simulink model "Final_proj"  (R2019a)
settings: Solver=VariableStepAuto  StartTime=0.0  StopTime=300  RelTol=1e-3
undefined symbols (not defined in the file): A, b, B, c, F, KI_, KT, KT_
settings Model: Creator=agtaye  LastModifiedBy=agtaye

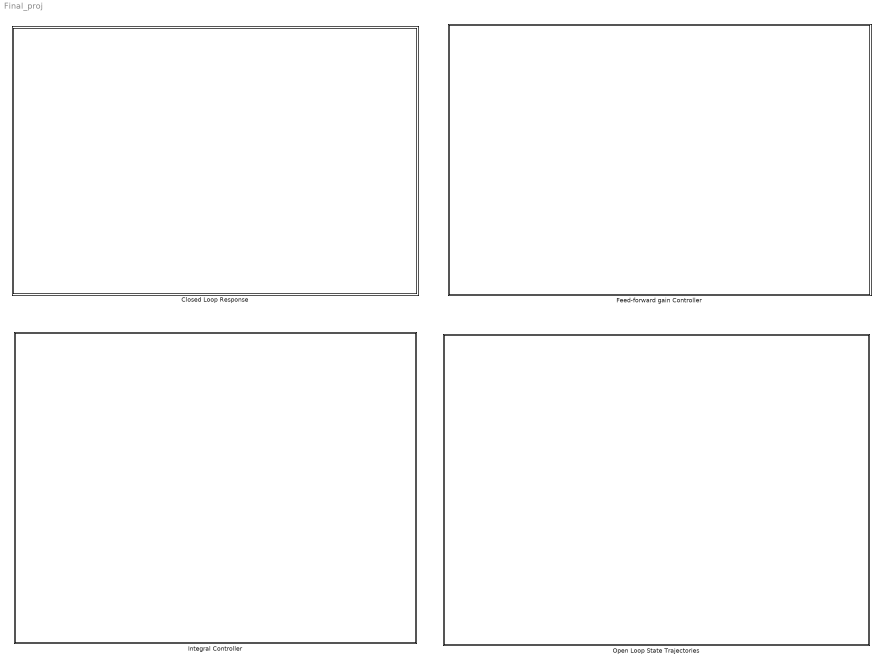
== system Final_proj ==
  Closed Loop Response : Subsystem
  Feed-forward gain Controller : Subsystem
  Integral Controller : Subsystem
  Open Loop State Trajectories : Subsystem

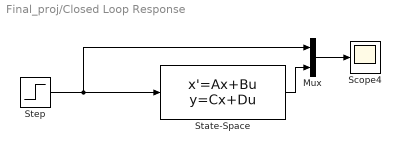
== system Final_proj/Closed Loop Response ==
  Mux : Mux  Inputs=2
  Scope4 : Scope
  State-Space : StateSpace  A="[0\t1\t0\t0; 63.7929491356160\t-5.61041746387390\t-70.7129377085583\t5.60838779731902; 46.9375000000000\t0\t-48.1712500000000\t1; 2182.58450488262\t-49.4418039003888\t-2245.08904324417\t50.6576674638739]"  B=[0;0.0006;0;0.0056]  C=[0 0 1 0]  D=0  InitialCondition=0
  Step : Step  Time=0  After=2  SampleTime=0
  wires:
  Mux/1 -> Scope4/1
  Step/1 -> Mux/1, State-Space/1
  State-Space/1 -> Mux/2

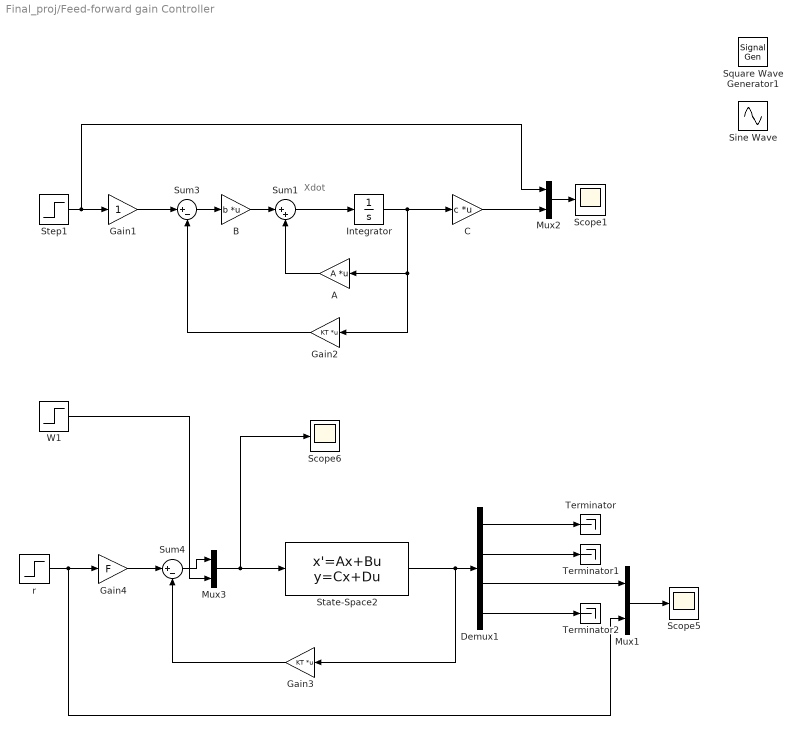
== system Final_proj/Feed-forward gain Controller ==
  note: Xdot
  A : Gain  Gain=A  Multiplication=Matrix(K*u)
  B : Gain  Gain=b  Multiplication=Matrix(K*u)
  "C " : Gain  Gain=c  Multiplication=Matrix(K*u)
  Demux1 : Demux
  Gain1 : Gain
  Gain2 : Gain  Gain=KT  Multiplication=Matrix(K*u)
  Gain3 : Gain  Gain=KT  Multiplication=Matrix(K*u)
  Gain4 : Gain  Gain=F
  Integrator : Integrator
  Mux1 : Mux  Inputs=2
  Mux2 : Mux  Inputs=2
  Mux3 : Mux  Inputs=2
  Scope1 : Scope
  Scope5 : Scope
  Scope6 : Scope
  Sine Wave : Sin  Amplitude=0.00001  Frequency=0.05  SampleTime=0
  Square Wave Generator1 : SignalGenerator  WaveForm=square  Amplitude=0.00001  Frequency=0.05  Units=rad/sec
  State-Space2 : StateSpace  A=A  B=B  C=eye(4)  D=[0 0;0 0;0 0;0 0]  InitialCondition=0
  Step1 : Step  Time=0  After=2  SampleTime=0
  Sum1 : Sum  Inputs=|++
  Sum3 : Sum  Inputs=|+-
  Sum4 : Sum  Inputs=|+-
  Terminator : Terminator
  Terminator1 : Terminator
  Terminator2 : Terminator
  W1 : Step  Time=10  After=0  SampleTime=0
  r : Step  Time=0  After=2  SampleTime=0
  wires:
  State-Space2/1 -> Demux1/1, Gain3/1
  Gain4/1 -> Sum4/1
  Gain3/1 -> Sum4/2
  Sum1/1 -> Integrator/1
  Integrator/1 -> "C "/1, Gain2/1, A/1
  Demux1/2 -> Terminator1/1
  A/1 -> Sum1/2
  Demux1/1 -> Terminator/1
  r/1 -> Gain4/1, Mux1/2
  Gain2/1 -> Sum3/2
  Sum4/1 -> Mux3/1
  Step1/1 -> Mux2/1, Gain1/1
  Gain1/1 -> Sum3/1
  B/1 -> Sum1/1
  Demux1/4 -> Terminator2/1
  Sum3/1 -> B/1
  Mux3/1 -> Scope6/1, State-Space2/1
  "C "/1 -> Mux2/2
  Mux2/1 -> Scope1/1
  Demux1/3 -> Mux1/1
  Mux1/1 -> Scope5/1
  W1/1 -> Mux3/2

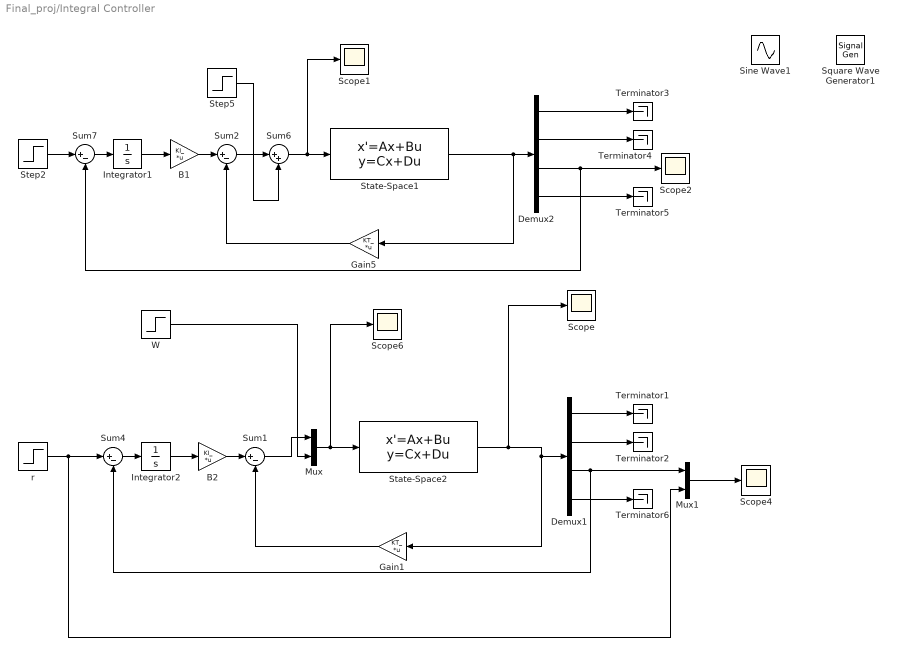
== system Final_proj/Integral Controller ==
  B1 : Gain  Gain=KI_  Multiplication=Matrix(K*u)
  B2 : Gain  Gain=KI_  Multiplication=Matrix(K*u)
  Demux1 : Demux
  Demux2 : Demux
  Gain1 : Gain  Gain=KT_  Multiplication=Matrix(K*u)
  Gain5 : Gain  Gain=KT_  Multiplication=Matrix(K*u)
  Integrator1 : Integrator
  Integrator2 : Integrator
  Mux : Mux  Inputs=2
  Mux1 : Mux  Inputs=2
  Scope{,1..2,4,6} (5 alike) : Scope
  Sine Wave1 : Sin  Amplitude=0.00001  Frequency=0.05  SampleTime=0
  Square Wave Generator1 : SignalGenerator  WaveForm=square  Amplitude=0.00001  Frequency=0.05  Units=rad/sec
  State-Space1 : StateSpace  A=A  B=b  C=eye(4)  D=[0;0;0;0]  InitialCondition=0
  State-Space2 : StateSpace  A=A  B=B  C=eye(4)  D=[0 0;0 0;0 0;0 0]  InitialCondition=0
  Step2 : Step  Time=0  After=2  SampleTime=0
  Step5 : Step  Time=10  SampleTime=0
  Sum{1..2,4,7} (4 alike) : Sum  Inputs=|+-
  Sum6 : Sum  Inputs=|++
  Terminator{1..6} (6 alike) : Terminator
  W : Step  Time=10  After=0.00001  SampleTime=0
  r : Step  Time=0  After=2  SampleTime=0
  wires:
  Demux2/3 -> Sum7/2, Scope2/1
  Gain5/1 -> Sum2/2
  Demux2/1 -> Terminator3/1
  Step2/1 -> Sum7/1
  State-Space1/1 -> Gain5/1, Demux2/1
  Sum6/1 -> Scope1/1, State-Space1/1
  B1/1 -> Sum2/1
  Integrator1/1 -> B1/1
  Sum2/1 -> Sum6/1
  Demux2/4 -> Terminator5/1
  Demux2/2 -> Terminator4/1
  Sum7/1 -> Integrator1/1
  Step5/1 -> Sum6/2
  Sum4/1 -> Integrator2/1
  Demux1/2 -> Terminator2/1
  Demux1/4 -> Terminator6/1
  Sum1/1 -> Mux/1
  Integrator2/1 -> B2/1
  B2/1 -> Sum1/1
  Mux/1 -> Scope6/1, State-Space2/1
  State-Space2/1 -> Scope/1, Demux1/1, Gain1/1
  r/1 -> Sum4/1, Mux1/2
  Demux1/1 -> Terminator1/1
  Gain1/1 -> Sum1/2
  Demux1/3 -> Mux1/1, Sum4/2
  Mux1/1 -> Scope4/1
  W/1 -> Mux/2

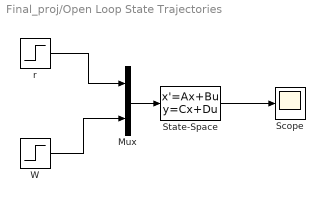
== system Final_proj/Open Loop State Trajectories ==
  Mux : Mux  Inputs=2
  Scope : Scope
  State-Space : StateSpace  A=A  B=B  C=eye(4)  D=[0 0;0 0;0 0;0 0]  InitialCondition=0
  W : Step  Time=0  After=0  SampleTime=0
  r : Step  Time=0  SampleTime=0
  wires:
  W/1 -> Mux/2
  State-Space/1 -> Scope/1
  Mux/1 -> State-Space/1
  r/1 -> Mux/1
